simulink model "DoublePulseTest"  (R2018a)
settings: Solver=FixedStepDiscrete  StartTime=0.0  StopTime=60e-6  RelTol=1e-3
values from neighbouring files (symbols this model uses):
  Cdg = 30e-12    (= 3e-11)    [sim_param.m]
  Cgs = 910e-12    (= 9.1e-10)    [sim_param.m]
  D = 0.5    [sim_param.m]
  Lg = 30e-9    (= 3e-08)    [sim_param.m]
  LLoad = 1e-3    (= 0.001)    [sim_param.m]
  Lss = 30e-9    (= 3e-08)    [sim_param.m]
  Rds = 0.1    [sim_param.m]
  Rg = 5    [sim_param.m]
  Vdc = 200    [sim_param.m]
  Vth = 3    [sim_param.m]
libraries: powerlib x17, pePwmGenerator x1
settings Model: Creator=enes_  LastModifiedBy=enes_

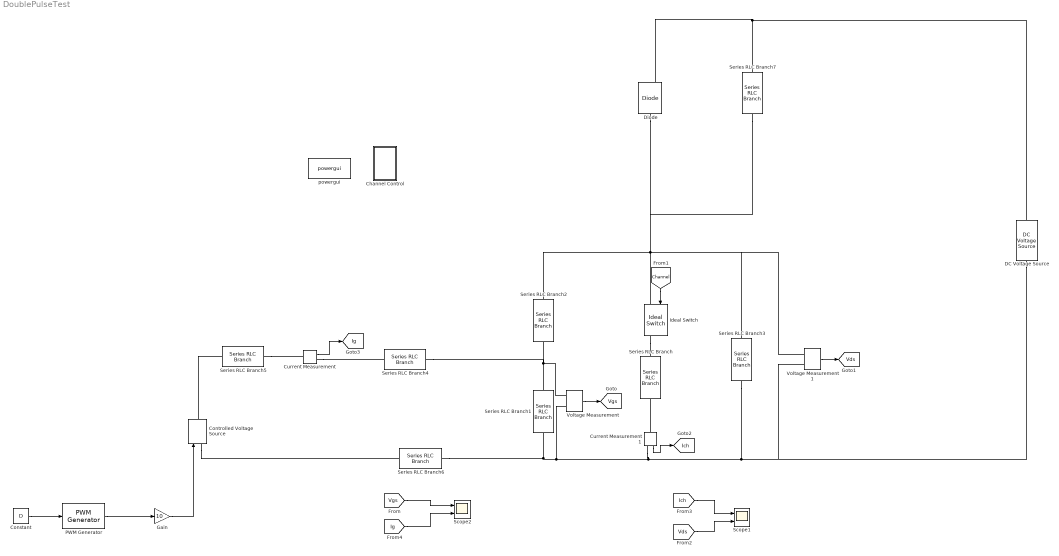
== system DoublePulseTest ==
  Channel Control : Subsystem
  Constant : Constant  Value=D
  Controlled Voltage Source : powerlib/Electrical Sources/Controlled Voltage Source  Initialize=on  Source_Type=AC  Amplitude=0  Phase=0  Frequency=0  Measurements=None
  Current Measurement : powerlib/Measurements/Current Measurement  PhasorSimulation=off  OutputType=Complex  PSBequivalent=0
  Current Measurement1 : powerlib/Measurements/Current Measurement  PhasorSimulation=off  OutputType=Complex  PSBequivalent=0
  DC Voltage Source : powerlib/Electrical Sources/DC Voltage Source  Amplitude=Vdc  Measurements=None
  Diode : powerlib/Power Electronics/Diode  Ron=0.001  Lon=0  Vf=0.8  IC=0  UseSnubber=0  Rs=500  Cs=250e-9  Measurements=on
  Gain : Gain  Gain=10
  Ideal Switch : powerlib/Power Electronics/Ideal Switch  Ron=0.001  Lon=0  IC=0  Rs=1e5  Cs=inf  Measurements=on
  PWM Generator : pePwmGenerator/PWM Generator  CarrCount=Up  Tper=20e-6  Ts=1e-7
  Scope1 : Scope  NumInputPorts=2
  Scope2 : Scope  NumInputPorts=2
  Series RLC Branch : powerlib/Elements/Series RLC Branch  LConnTagsString=__new0  RConnTagsString=__new0  BranchType=R  Resistance=Rds  Inductance=1e-3  SetiL0=off  InitialCurrent=0  Capacitance=1e-6  Setx0=off  InitialVoltage=0  Measurements=None
  Series RLC Branch1 : powerlib/Elements/Series RLC Branch  LConnTagsString=__new0  RConnTagsString=__new0  BranchType=C  Resistance=Rds  Inductance=1e-3  SetiL0=off  InitialCurrent=0  Capacitance=Cgs  Setx0=off  InitialVoltage=0  Measurements=None
  Series RLC Branch2 : powerlib/Elements/Series RLC Branch  LConnTagsString=__new0  RConnTagsString=__new0  BranchType=C  Resistance=Rds  Inductance=1e-3  SetiL0=off  InitialCurrent=0  Capacitance=Cdg  Setx0=off  InitialVoltage=0  Measurements=None
  Series RLC Branch3 : powerlib/Elements/Series RLC Branch  LConnTagsString=__new0  RConnTagsString=__new0  BranchType=C  Resistance=Rds  Inductance=1e-3  SetiL0=off  InitialCurrent=0  Capacitance=Cdg  Setx0=off  InitialVoltage=0  Measurements=None
  Series RLC Branch4 : powerlib/Elements/Series RLC Branch  LConnTagsString=__new0  RConnTagsString=__new0  BranchType=R  Resistance=Rg  Inductance=1e-3  SetiL0=off  InitialCurrent=0  Capacitance=1e-6  Setx0=off  InitialVoltage=0  Measurements=None
  Series RLC Branch5 : powerlib/Elements/Series RLC Branch  LConnTagsString=__new0  RConnTagsString=__new0  BranchType=L  Resistance=Rg  Inductance=Lg  SetiL0=off  InitialCurrent=0  Capacitance=1e-6  Setx0=off  InitialVoltage=0  Measurements=None
  Series RLC Branch6 : powerlib/Elements/Series RLC Branch  LConnTagsString=__new0  RConnTagsString=__new0  BranchType=L  Resistance=Rg  Inductance=Lss  SetiL0=off  InitialCurrent=0  Capacitance=1e-6  Setx0=off  InitialVoltage=0  Measurements=None
  Series RLC Branch7 : powerlib/Elements/Series RLC Branch  LConnTagsString=__new0  RConnTagsString=__new0  BranchType=L  Resistance=Rg  Inductance=LLoad  SetiL0=off  InitialCurrent=0  Capacitance=1e-6  Setx0=off  InitialVoltage=0  Measurements=None
  Voltage Measurement : powerlib/Measurements/Voltage Measurement  PhasorSimulation=off  OutputType=Complex  PSBequivalent=0
  Voltage Measurement1 : powerlib/Measurements/Voltage Measurement  PhasorSimulation=off  OutputType=Complex  PSBequivalent=0
  powergui : powerlib/powergui  Priority=1  SimulationMode=Discrete  SampleTime=1e-12  frequency=60  Iterations=50  frequencyindice=0  Pbase=100e6  ErrMax=1e-4  UnitsV=kV  UnitsW=MW  buscounter=0  FunctionMessages=off  echomessages=off  EnableUseOfTLC=off  CurrentSourceSwitches=off  DisableSnubberDevices=off  DisableRonSwitches=off  DisableVfSwitches=off  DisplayEquations=off  SolverType=Tustin/Backward Euler (TBE)  Interpol=off  ExternalGateDelay=off  methode=off  Ts=100  x0status=blocks  SPID=on  SwTol=0  HookPort=off  RestoreLinks=warning  ResistiveCurrentMeasurement=off  Frange=[0:2:500]  Ylog=off  Xlog=on  ShowGrid=off  save=off  variable=ZData  structure=0  ZoomFFT=off  StartTime=0.0  cycles=1  DisplayStyle=1  fundamental=60  FreqAxis=off  MaxFrequency=1000  frequencyindicesteady=1  RmsSteady=1  display=off
  tag scope: Ich=global, Ig=global, Vds=global, Vgs=global
  wires:
  Voltage Measurement/1 -> [Vgs]
  [Channel] -> Ideal Switch/1
  PWM Generator/1 -> Gain/1
  Constant/1 -> PWM Generator/1
  Gain/1 -> Controlled Voltage Source/1
  [Vgs] -> Scope2/1
  Voltage Measurement1/1 -> [Vds]
  Current Measurement1/1 -> [Ich]
  [Ich] -> Scope1/1
  [Vds] -> Scope1/2
  Current Measurement/1 -> [Ig]
  [Ig] -> Scope2/2
  connections:
  Ideal Switch/RConn1 -- Series RLC Branch/LConn1
  Ideal Switch/LConn1 -- Series RLC Branch3/LConn1 -- Voltage Measurement1/LConn1 -- Series RLC Branch7/RConn1 -- Diode/LConn1 -- Series RLC Branch2/LConn1
  Series RLC Branch1/LConn1 -- Series RLC Branch4/RConn1 -- Series RLC Branch2/RConn1 -- Voltage Measurement/LConn1
  Series RLC Branch3/RConn1 -- Voltage Measurement1/LConn2 -- DC Voltage Source/LConn1 -- Current Measurement1/RConn1 -- Series RLC Branch6/RConn1 -- Series RLC Branch1/RConn1 -- Voltage Measurement/LConn2
  Current Measurement/RConn1 -- Series RLC Branch4/LConn1
  Series RLC Branch5/RConn1 -- Current Measurement/LConn1
  Controlled Voltage Source/RConn1 -- Series RLC Branch5/LConn1
  Controlled Voltage Source/LConn1 -- Series RLC Branch6/LConn1
  Series RLC Branch7/LConn1 -- DC Voltage Source/RConn1 -- Diode/RConn1
  Current Measurement1/LConn1 -- Series RLC Branch/RConn1

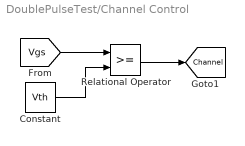
== system DoublePulseTest/Channel Control ==
  Constant : Constant  Value=Vth
  Relational Operator : RelationalOperator  OutDataTypeStr=boolean  RndMeth=Simplest
  tag scope: Channel=global
  wires:
  [Vgs] -> Relational Operator/1
  Relational Operator/1 -> [Channel]
  Constant/1 -> Relational Operator/2
